simulink model "snap2_f_200msps_64i_4096c"  (R2019a)
settings: Solver=VariableStepDiscrete  StartTime=0.0  StopTime=10.0  RelTol=1e-3
undefined symbols (not defined in the file or in its folder): datetime, posixtime
libraries: xbsIndex_r4 x21354, casper_library_misc x297, casper_library_delays x19, xps_library x14, casper_library_sources x4
(part 5 of 217)

== system snap2_f_200msps_64i_4096c/input ==
  adc : Inport
  noise : Inport  Port=2
  sync : Inport  Port=3
  Constant4 : xbsIndex_r4/Constant  const=0  gui_display_data_type=Fixed-point  arith_type=Unsigned  n_bits=10*64  bin_pt=0  preci_type=Single  exp_width=8  frac_width=24  explicit_period=on  period=1  equ=P=C  opselect=C  inp2=PCIN>>17  opr=+  inp1=P  carry=CIN  dbl_ovrd=off  block_type=constant
  bit_stats : Subsystem
  bus_create2 : Subsystem  AncestorBlock=casper_library_flow_control/bus_create  mask(bus_create){inputNum=4}
      mask prompts: inputNum "Number of inputs:"
      mask init:
      | bus_create_init(gcb,...
      |     'inputNum', inputNum);
  bus_mux : Subsystem  AncestorBlock=casper_library_bus/bus_mux  mask(bus_mux){n_inputs=4, n_bits=10 * ones(64,1), cmplx=off, misc=on, mux_latency=1}
      mask prompts: n_inputs "number of inputs"; n_bits "input bit widths"; cmplx "complex data"; misc "misc support"; mux_latency "mux latency"
      mask help: Mux components of bus
      mask init:
      | bus_mux_init(gcb, ...
      |     'n_inputs', n_inputs, ...
      |     'n_bits', n_bits, ...
      |     'cmplx', cmplx, ...
      |     'misc', misc, ...
      |     'mux_latency', mux_latency);
  counter_test_signal : Subsystem
  rms : Subsystem
  slice3 : xbsIndex_r4/Slice  nbits=2*64  boolean_output=off  mode=Lower Bit Location + Width  bit1=0  base1=MSB of Input  bit0=0  base0=LSB of Input  dbl_ovrd=off  block_type=slice
  source_sel0 : Subsystem  Tag=xps:sw_reg  AncestorBlock=xps_library/Memory/software_register  mask(swreg){io_dir=From Processor, io_delay=0, init_val=0, sample_period=1, names=reg, bitwidths=32, bin_pts=0, arith_types=0, sim_port=on, show_format=off, desc_str=|}
      mask desc_str=|
      | Selector control to determine if signal streams carry
      | ADC samples, digital noise samples, or zeros.
      | Streams ``n=0..15`` is controlled by register
      | bits ``[2n+1:2n]``. Value ``0`` selects noise;
      | ``1`` selects ADC; ``2`` selects zeros.
      mask prompts: io_dir "I/O direction"; io_delay "I/O delay"; init_val "Initial Value"; sample_period "Sample period"; names "Bitfield names [msb...lsb]"; bitwidths "Bitfield widths"; bin_pts "Bitfield binary pts"; arith_types "Bitfield types, ufix=0, fix=1, bool=2"; sim_port "Provide sim input/output?"; show_format "Print format string?"; desc_str "Description"
      mask help: A 32-bit software-accessible register. Can be divided into bitfields of varying widths and types using the fields in the block mask.
      mask init:
      | swreg_init(gcb)
      settings: AttributesFormatString=1input
      mask TypeOptions io_dir: To Processor | From Processor
      mask Callback io_dir:
      | mask_enables = get_param(gcb, 'MaskEnables');
      | mask_names = get_param(gcb, 'MaskNames');
      | if strcmp(get_param(gcb, 'io_dir'), 'To Processor'),
      |     mask_enables{ismember(mask_names, 'sample_period')} = 'off';
      | else
      |     mask_enables{ismember(mask_names, 'sample_period')} = 'on';
      | end
      | set_param(gcb, 'MaskEnables', mask_enables);
      mask DialogControl ParameterTabVar0 Prompt: Setup
  source_sel1 : Subsystem  Tag=xps:sw_reg  AncestorBlock=xps_library/Memory/software_register  mask(swreg){io_dir=From Processor, io_delay=0, init_val=0, sample_period=1, names=reg, bitwidths=32, bin_pts=0, arith_types=0, sim_port=on, show_format=off, desc_str=|}
      mask desc_str=|
      | Selector control to determine if signal streams carry
      | ADC samples, digital noise samples, or zeros.
      | Streams ``n=16..31`` is controlled by register
      | bits ``[2(n-16)+1:2(n-16)]``. Value ``0`` selects noise;
      | ``1`` selects ADC; ``2`` selects zeros.
      mask prompts: io_dir "I/O direction"; io_delay "I/O delay"; init_val "Initial Value"; sample_period "Sample period"; names "Bitfield names [msb...lsb]"; bitwidths "Bitfield widths"; bin_pts "Bitfield binary pts"; arith_types "Bitfield types, ufix=0, fix=1, bool=2"; sim_port "Provide sim input/output?"; show_format "Print format string?"; desc_str "Description"
      mask help: A 32-bit software-accessible register. Can be divided into bitfields of varying widths and types using the fields in the block mask.
      mask init:
      | swreg_init(gcb)
      settings: AttributesFormatString=1input
      mask TypeOptions io_dir: To Processor | From Processor
      mask Callback io_dir:
      | mask_enables = get_param(gcb, 'MaskEnables');
      | mask_names = get_param(gcb, 'MaskNames');
      | if strcmp(get_param(gcb, 'io_dir'), 'To Processor'),
      |     mask_enables{ismember(mask_names, 'sample_period')} = 'off';
      | else
      |     mask_enables{ismember(mask_names, 'sample_period')} = 'on';
      | end
      | set_param(gcb, 'MaskEnables', mask_enables);
      mask DialogControl ParameterTabVar0 Prompt: Setup
  source_sel2 : Subsystem  Tag=xps:sw_reg  AncestorBlock=xps_library/Memory/software_register  mask(swreg){io_dir=From Processor, io_delay=0, init_val=0, sample_period=1, names=reg, bitwidths=32, bin_pts=0, arith_types=0, sim_port=on, show_format=off, desc_str=|}
      mask desc_str=|
      | Selector control to determine if signal streams carry
      | ADC samples, digital noise samples, or zeros.
      | Streams ``n=32..47`` is controlled by register
      | bits ``[2(n-32)+1:2(n-32)]``. Value ``0`` selects noise;
      | ``1`` selects ADC; ``2`` selects zeros.
      mask prompts: io_dir "I/O direction"; io_delay "I/O delay"; init_val "Initial Value"; sample_period "Sample period"; names "Bitfield names [msb...lsb]"; bitwidths "Bitfield widths"; bin_pts "Bitfield binary pts"; arith_types "Bitfield types, ufix=0, fix=1, bool=2"; sim_port "Provide sim input/output?"; show_format "Print format string?"; desc_str "Description"
      mask help: A 32-bit software-accessible register. Can be divided into bitfields of varying widths and types using the fields in the block mask.
      mask init:
      | swreg_init(gcb)
      settings: AttributesFormatString=1input
      mask TypeOptions io_dir: To Processor | From Processor
      mask Callback io_dir:
      | mask_enables = get_param(gcb, 'MaskEnables');
      | mask_names = get_param(gcb, 'MaskNames');
      | if strcmp(get_param(gcb, 'io_dir'), 'To Processor'),
      |     mask_enables{ismember(mask_names, 'sample_period')} = 'off';
      | else
      |     mask_enables{ismember(mask_names, 'sample_period')} = 'on';
      | end
      | set_param(gcb, 'MaskEnables', mask_enables);
      mask DialogControl ParameterTabVar0 Prompt: Setup
  source_sel3 : Subsystem  Tag=xps:sw_reg  AncestorBlock=xps_library/Memory/software_register  mask(swreg){io_dir=From Processor, io_delay=0, init_val=0, sample_period=1, names=reg, bitwidths=32, bin_pts=0, arith_types=0, sim_port=on, show_format=off, desc_str=|}
      mask desc_str=|
      | Selector control to determine if signal streams carry
      | ADC samples, digital noise samples, or zeros.
      | Streams ``n=48..63`` is controlled by register
      | bits ``[2(n-48)+1:2(n-48)]``. Value ``0`` selects noise;
      | ``1`` selects ADC; ``2`` selects zeros.
      mask prompts: io_dir "I/O direction"; io_delay "I/O delay"; init_val "Initial Value"; sample_period "Sample period"; names "Bitfield names [msb...lsb]"; bitwidths "Bitfield widths"; bin_pts "Bitfield binary pts"; arith_types "Bitfield types, ufix=0, fix=1, bool=2"; sim_port "Provide sim input/output?"; show_format "Print format string?"; desc_str "Description"
      mask help: A 32-bit software-accessible register. Can be divided into bitfields of varying widths and types using the fields in the block mask.
      mask init:
      | swreg_init(gcb)
      settings: AttributesFormatString=1input
      mask TypeOptions io_dir: To Processor | From Processor
      mask Callback io_dir:
      | mask_enables = get_param(gcb, 'MaskEnables');
      | mask_names = get_param(gcb, 'MaskNames');
      | if strcmp(get_param(gcb, 'io_dir'), 'To Processor'),
      |     mask_enables{ismember(mask_names, 'sample_period')} = 'off';
      | else
      |     mask_enables{ismember(mask_names, 'sample_period')} = 'on';
      | end
      | set_param(gcb, 'MaskEnables', mask_enables);
      mask DialogControl ParameterTabVar0 Prompt: Setup
  sync_out : Outport
  dout : Outport  Port=2
  wires:
  Constant4/1 -> bus_mux/4(d2)
  sync/1 -> bus_mux/6(misci)
  bus_mux/1(out) -> dout/1, bit_stats/1(din), rms/1(in)
  slice3/1 -> bus_mux/1(sel)
  adc/1 -> bus_mux/3(d1)
  noise/1 -> bus_mux/2(d0)
  bus_mux/2(misco) -> sync_out/1
  source_sel1/1(in_reg) -> bus_create2/2(in2)
  source_sel0/1(in_reg) -> bus_create2/1(in1)
  source_sel2/1(in_reg) -> bus_create2/3(in3)
  bus_create2/1(bus_out) -> slice3/1
  source_sel3/1(in_reg) -> bus_create2/4(in4)
  counter_test_signal/1(Out1) -> bus_mux/5(d3)

== system snap2_f_200msps_64i_4096c/mask ==
  note: accumulation length in spectra
  note: delay by 2 so new_acc precedes
      | first spectra of a new accumulation.
      | 1 cycle for tt_counter load.
      | 1 cycle for target_tt compare
  note: starts on 1
  sync : Inport
  din : Inport  Port=2
  tt : Inport  Port=3
  Concat : xbsIndex_r4/Concat  num_inputs=2  dbl_ovrd=off  block_type=concat
  Constant : Constant  Value=8192*2
  Constant1 : Constant  Value=0
  Constant2 : Constant  Value=3
  Constant3 : Constant  Value=10
  Counter : xbsIndex_r4/Counter  cnt_type=Free Running  cnt_to=Inf  operation=Up  start_count=1  cnt_by_val=1  arith_type=Unsigned  n_bits=32  bin_pt=0  load_pin=off  rst=on  en=off  explicit_period=on  period=1  use_behavioral_HDL=off  implementation=Fabric  dbl_ovrd=off  block_type=counter
  Counter1 : xbsIndex_r4/Counter  cnt_type=Free Running  cnt_to=Inf  operation=Up  start_count=0  cnt_by_val=1  arith_type=Unsigned  n_bits=32  bin_pt=0  load_pin=off  rst=off  en=on  explicit_period=on  period=1  use_behavioral_HDL=off  implementation=Fabric  dbl_ovrd=off  block_type=counter
  Delay{,1..7} (8 alike) : xbsIndex_r4/Delay  rst=off  infoeditControl=Selection of Reset will increase slice count due to use of real FFs and instead of SRLs  en=off  latency=2  reg_retiming=on  dbl_ovrd=off  block_type=delay
  Delay8 : xbsIndex_r4/Delay  rst=off  infoeditControl=Selection of Reset will increase slice count due to use of real FFs and instead of SRLs  en=off  latency=1  reg_retiming=on  dbl_ovrd=off  block_type=delay
  Logical : xbsIndex_r4/Logical  logical_function=OR  inputs=2  en=off  latency=0  precision=Full  arith_type=Unsigned  n_bits=16  bin_pt=0  align_bp=on  dbl_ovrd=off  block_type=logical
  Register : xbsIndex_r4/Register  init=0  rst=off  en=on  dbl_ovrd=off  block_type=register
  Reinterpret : xbsIndex_r4/Reinterpret  force_arith_type=off  arith_type=Unsigned  force_bin_pt=on  bin_pt=18  block_type=reinterpret
  Relational : xbsIndex_r4/Relational  mode=a=b  op_type=Bool  en=off  latency=1  dbl_ovrd=off  block_type=relational
  Relational1 : xbsIndex_r4/Relational  mode=a=b  op_type=Bool  en=off  latency=0  dbl_ovrd=off  block_type=relational
  Slice : xbsIndex_r4/Slice  nbits=32-(nfft_bits - 3 + ninput_bits - 2)  boolean_output=off  mode=Lower Bit Location + Width  bit1=0  base1=MSB of Input  bit0=nfft_bits - 3 + ninput_bits - 2  base0=LSB of Input  dbl_ovrd=off  block_type=slice
  acc_cnt : Subsystem  Tag=xps:sw_reg  AncestorBlock=xps_library/Memory/software_register  mask(swreg){io_dir=To Processor, io_delay=0, init_val=0, sample_period=1, names=reg, bitwidths=32, bin_pts=0, arith_types=0, sim_port=on, show_format=on, desc_str=""}
      mask prompts: io_dir "I/O direction"; io_delay "I/O delay"; init_val "Initial Value"; sample_period "Sample period"; names "Bitfield names [msb...lsb]"; bitwidths "Bitfield widths"; bin_pts "Bitfield binary pts"; arith_types "Bitfield types, ufix=0, fix=1, bool=2"; sim_port "Provide sim input/output?"; show_format "Print format string?"; desc_str "Description"
      mask help: A 32-bit software-accessible register. Can be divided into bitfields of varying widths and types using the fields in the block mask.
      mask init:
      | swreg_init(gcb)
      settings: AttributesFormatString=1output:uf32.0 = 32 bits
      mask TypeOptions io_dir: To Processor | From Processor
      mask Callback io_dir:
      | mask_enables = get_param(gcb, 'MaskEnables');
      | mask_names = get_param(gcb, 'MaskNames');
      | if strcmp(get_param(gcb, 'io_dir'), 'To Processor'),
      |     mask_enables{ismember(mask_names, 'sample_period')} = 'off';
      | else
      |     mask_enables{ismember(mask_names, 'sample_period')} = 'on';
      | end
      | set_param(gcb, 'MaskEnables', mask_enables);
      mask DialogControl ParameterTabVar0 Prompt: Setup
  acc_len : Subsystem  Tag=xps:sw_reg  AncestorBlock=xps_library/Memory/software_register  mask(swreg){io_dir=From Processor, io_delay=0, init_val=0, sample_period=1, names=reg, bitwidths=32, bin_pts=0, arith_types=0, sim_port=on, show_format=on, desc_str=""}
      mask prompts: io_dir "I/O direction"; io_delay "I/O delay"; init_val "Initial Value"; sample_period "Sample period"; names "Bitfield names [msb...lsb]"; bitwidths "Bitfield widths"; bin_pts "Bitfield binary pts"; arith_types "Bitfield types, ufix=0, fix=1, bool=2"; sim_port "Provide sim input/output?"; show_format "Print format string?"; desc_str "Description"
      mask help: A 32-bit software-accessible register. Can be divided into bitfields of varying widths and types using the fields in the block mask.
      mask init:
      | swreg_init(gcb)
      settings: AttributesFormatString=1input:uf32.0 = 32 bits
      mask TypeOptions io_dir: To Processor | From Processor
      mask Callback io_dir:
      | mask_enables = get_param(gcb, 'MaskEnables');
      | mask_names = get_param(gcb, 'MaskNames');
      | if strcmp(get_param(gcb, 'io_dir'), 'To Processor'),
      |     mask_enables{ismember(mask_names, 'sample_period')} = 'off';
      | else
      |     mask_enables{ismember(mask_names, 'sample_period')} = 'on';
      | end
      | set_param(gcb, 'MaskEnables', mask_enables);
      mask DialogControl ParameterTabVar0 Prompt: Setup
  acc_time_lsb : Subsystem  Tag=xps:sw_reg  AncestorBlock=xps_library/Memory/software_register  mask(swreg){io_dir=To Processor, io_delay=0, init_val=0, sample_period=1, names=reg, bitwidths=32, bin_pts=0, arith_types=0, sim_port=on, show_format=on, desc_str=""}
      mask prompts: io_dir "I/O direction"; io_delay "I/O delay"; init_val "Initial Value"; sample_period "Sample period"; names "Bitfield names [msb...lsb]"; bitwidths "Bitfield widths"; bin_pts "Bitfield binary pts"; arith_types "Bitfield types, ufix=0, fix=1, bool=2"; sim_port "Provide sim input/output?"; show_format "Print format string?"; desc_str "Description"
      mask help: A 32-bit software-accessible register. Can be divided into bitfields of varying widths and types using the fields in the block mask.
      mask init:
      | swreg_init(gcb)
      settings: AttributesFormatString=1output:uf32.0 = 32 bits
      mask TypeOptions io_dir: To Processor | From Processor
      mask Callback io_dir:
      | mask_enables = get_param(gcb, 'MaskEnables');
      | mask_names = get_param(gcb, 'MaskNames');
      | if strcmp(get_param(gcb, 'io_dir'), 'To Processor'),
      |     mask_enables{ismember(mask_names, 'sample_period')} = 'off';
      | else
      |     mask_enables{ismember(mask_names, 'sample_period')} = 'on';
      | end
      | set_param(gcb, 'MaskEnables', mask_enables);
      mask DialogControl ParameterTabVar0 Prompt: Setup
  acc_time_msb : Subsystem  Tag=xps:sw_reg  AncestorBlock=xps_library/Memory/software_register  mask(swreg){io_dir=To Processor, io_delay=0, init_val=0, sample_period=1, names=reg, bitwidths=32, bin_pts=0, arith_types=0, sim_port=on, show_format=on, desc_str=""}
      mask prompts: io_dir "I/O direction"; io_delay "I/O delay"; init_val "Initial Value"; sample_period "Sample period"; names "Bitfield names [msb...lsb]"; bitwidths "Bitfield widths"; bin_pts "Bitfield binary pts"; arith_types "Bitfield types, ufix=0, fix=1, bool=2"; sim_port "Provide sim input/output?"; show_format "Print format string?"; desc_str "Description"
      mask help: A 32-bit software-accessible register. Can be divided into bitfields of varying widths and types using the fields in the block mask.
      mask init:
      | swreg_init(gcb)
      settings: AttributesFormatString=1output:uf32.0 = 32 bits
      mask TypeOptions io_dir: To Processor | From Processor
      mask Callback io_dir:
      | mask_enables = get_param(gcb, 'MaskEnables');
      | mask_names = get_param(gcb, 'MaskNames');
      | if strcmp(get_param(gcb, 'io_dir'), 'To Processor'),
      |     mask_enables{ismember(mask_names, 'sample_period')} = 'off';
      | else
      |     mask_enables{ismember(mask_names, 'sample_period')} = 'on';
      | end
      | set_param(gcb, 'MaskEnables', mask_enables);
      mask DialogControl ParameterTabVar0 Prompt: Setup
  bus_create2 : Subsystem  AncestorBlock=casper_library_flow_control/bus_create  mask(bus_create){inputNum=4}
      mask prompts: inputNum "Number of inputs:"
      mask init:
      | bus_create_init(gcb,...
      |     'inputNum', inputNum);
  bus_expand : Subsystem  AncestorBlock=casper_library_flow_control/bus_expand  mask(bus_expand){mode=divisions of equal size, outputNum=2, outputWidth=32, outputBinaryPt=0, outputArithmeticType=0, show_format=off, outputToWorkspace=off, variablePrefix=out, outputToModelAsWell=on}
      mask prompts: outputNum "Number of outputs:"; outputWidth "Output width:"; outputBinaryPt "Output binary point position:"; outputArithmeticType "Output arithmetic type (ufix=0, fix=1, bool=2):"; show_format "Print format string?"; outputToWorkspace "Output to workspace?"; variablePrefix "Variable name prefix:"; outputToModelAsWell "Output to model as well?"
      mask help:
      | Expands a 'bus' made using a bus_create or Xilinx
      | concat block.
      | The input will be divided into the specified number
      | of outputs with the specified arithmetic types.
      | Divisions are made from most significant bit.
      mask init: same as snap2_f_200msps_64i_4096c/autocorr/bus_expand
      settings: AttributesFormatString=2 outputs
      mask TypeOptions mode: divisions of equal size | divisions of arbitrary size
      mask Callback mode: bus_expand_callback();
      mask Callback outputWidth: bus_expand_callback();
      mask Callback outputToWorkspace: bus_expand_callback();
  bus_expand4 : Subsystem  AncestorBlock=casper_library_flow_control/bus_expand  mask(bus_expand){mode=divisions of equal size, outputNum=4, outputWidth=36*8, outputBinaryPt=0, outputArithmeticType=0, show_format=off, outputToWorkspace=off, variablePrefix=out, outputToModelAsWell=on}
      mask prompts: outputNum "Number of outputs:"; outputWidth "Output width:"; outputBinaryPt "Output binary point position:"; outputArithmeticType "Output arithmetic type (ufix=0, fix=1, bool=2):"; show_format "Print format string?"; outputToWorkspace "Output to workspace?"; variablePrefix "Variable name prefix:"; outputToModelAsWell "Output to model as well?"
      mask help:
      | Expands a 'bus' made using a bus_create or Xilinx
      | concat block.
      | The input will be divided into the specified number
      | of outputs with the specified arithmetic types.
      | Divisions are made from most significant bit.
      mask init: same as snap2_f_200msps_64i_4096c/autocorr/bus_expand
      settings: AttributesFormatString=4 outputs
      mask TypeOptions mode: divisions of equal size | divisions of arbitrary size
      mask Callback mode: bus_expand_callback();
      mask Callback outputWidth: bus_expand_callback();
      mask Callback outputToWorkspace: bus_expand_callback();
  core0 : Subsystem  mask{nchan_bits=nfft_bits - 3, ninput_bits=ninput_bits - 2, ram_latency=2}
      mask prompts: nchan_bits "Number of fft channels (2^?)"; ninput_bits "Number of Input signals (2^?)"; ram_latency "RAM latency"
  core1 : Subsystem  mask{nchan_bits=nfft_bits - 3, ninput_bits=ninput_bits - 2, ram_latency=2}
      mask prompts: nchan_bits "Number of fft channels (2^?)"; ninput_bits "Number of Input signals (2^?)"; ram_latency "RAM latency"
  core2 : Subsystem  mask{nchan_bits=nfft_bits - 3, ninput_bits=ninput_bits - 2, ram_latency=2}
      mask prompts: nchan_bits "Number of fft channels (2^?)"; ninput_bits "Number of Input signals (2^?)"; ram_latency "RAM latency"
  core3 : Subsystem  mask{nchan_bits=nfft_bits - 3, ninput_bits=ninput_bits - 2, ram_latency=2}
      mask prompts: nchan_bits "Number of fft channels (2^?)"; ninput_bits "Number of Input signals (2^?)"; ram_latency "RAM latency"
  target_tt_lsb : Subsystem  Tag=xps:sw_reg  AncestorBlock=xps_library/Memory/software_register  mask(swreg){io_dir=From Processor, io_delay=0, init_val=0, sample_period=1, names=reg, bitwidths=32, bin_pts=0, arith_types=0, sim_port=on, show_format=on, desc_str=""}
      mask prompts: io_dir "I/O direction"; io_delay "I/O delay"; init_val "Initial Value"; sample_period "Sample period"; names "Bitfield names [msb...lsb]"; bitwidths "Bitfield widths"; bin_pts "Bitfield binary pts"; arith_types "Bitfield types, ufix=0, fix=1, bool=2"; sim_port "Provide sim input/output?"; show_format "Print format string?"; desc_str "Description"
      mask help: A 32-bit software-accessible register. Can be divided into bitfields of varying widths and types using the fields in the block mask.
      mask init:
      | swreg_init(gcb)
      settings: AttributesFormatString=1input:uf32.0 = 32 bits
      mask TypeOptions io_dir: To Processor | From Processor
      mask Callback io_dir:
      | mask_enables = get_param(gcb, 'MaskEnables');
      | mask_names = get_param(gcb, 'MaskNames');
      | if strcmp(get_param(gcb, 'io_dir'), 'To Processor'),
      |     mask_enables{ismember(mask_names, 'sample_period')} = 'off';
      | else
      |     mask_enables{ismember(mask_names, 'sample_period')} = 'on';
      | end
      | set_param(gcb, 'MaskEnables', mask_enables);
      mask DialogControl ParameterTabVar0 Prompt: Setup
  target_tt_msb : Subsystem  Tag=xps:sw_reg  AncestorBlock=xps_library/Memory/software_register  mask(swreg){io_dir=From Processor, io_delay=0, init_val=0, sample_period=1, names=reg, bitwidths=32, bin_pts=0, arith_types=0, sim_port=on, show_format=on, desc_str=""}
      mask prompts: io_dir "I/O direction"; io_delay "I/O delay"; init_val "Initial Value"; sample_period "Sample period"; names "Bitfield names [msb...lsb]"; bitwidths "Bitfield widths"; bin_pts "Bitfield binary pts"; arith_types "Bitfield types, ufix=0, fix=1, bool=2"; sim_port "Provide sim input/output?"; show_format "Print format string?"; desc_str "Description"
      mask help: A 32-bit software-accessible register. Can be divided into bitfields of varying widths and types using the fields in the block mask.
      mask init:
      | swreg_init(gcb)
      settings: AttributesFormatString=1input:uf32.0 = 32 bits
      mask TypeOptions io_dir: To Processor | From Processor
      mask Callback io_dir:
      | mask_enables = get_param(gcb, 'MaskEnables');
      | mask_names = get_param(gcb, 'MaskNames');
      | if strcmp(get_param(gcb, 'io_dir'), 'To Processor'),
      |     mask_enables{ismember(mask_names, 'sample_period')} = 'off';
      | else
      |     mask_enables{ismember(mask_names, 'sample_period')} = 'on';
      | end
      | set_param(gcb, 'MaskEnables', mask_enables);
      mask DialogControl ParameterTabVar0 Prompt: Setup
  threshold : Subsystem  Tag=xps:sw_reg  AncestorBlock=xps_library/Memory/software_register  mask(swreg){io_dir=From Processor, io_delay=0, init_val=2^32 - 1, sample_period=1, names=reg, bitwidths=32, bin_pts=0, arith_types=0, sim_port=on, show_format=on, desc_str=""}
      mask prompts: io_dir "I/O direction"; io_delay "I/O delay"; init_val "Initial Value"; sample_period "Sample period"; names "Bitfield names [msb...lsb]"; bitwidths "Bitfield widths"; bin_pts "Bitfield binary pts"; arith_types "Bitfield types, ufix=0, fix=1, bool=2"; sim_port "Provide sim input/output?"; show_format "Print format string?"; desc_str "Description"
      mask help: A 32-bit software-accessible register. Can be divided into bitfields of varying widths and types using the fields in the block mask.
      mask init:
      | swreg_init(gcb)
      settings: AttributesFormatString=1input:uf32.0 = 32 bits
      mask TypeOptions io_dir: To Processor | From Processor
      mask Callback io_dir:
      | mask_enables = get_param(gcb, 'MaskEnables');
      | mask_names = get_param(gcb, 'MaskNames');
      | if strcmp(get_param(gcb, 'io_dir'), 'To Processor'),
      |     mask_enables{ismember(mask_names, 'sample_period')} = 'off';
      | else
      |     mask_enables{ismember(mask_names, 'sample_period')} = 'on';
      | end
      | set_param(gcb, 'MaskEnables', mask_enables);
      mask DialogControl ParameterTabVar0 Prompt: Setup
  tt_counter : xbsIndex_r4/Counter  cnt_type=Free Running  cnt_to=1  operation=Up  start_count=0  cnt_by_val=1  arith_type=Unsigned  n_bits=64  bin_pt=0  load_pin=on  rst=off  en=off  explicit_period=on  period=1  use_behavioral_HDL=off  implementation=Fabric  use_rpm=on  dbl_ovrd=off  block_type=counter
      settings: xl_area=[0, 0, 0, 0, 0, 0, 0]
  sync_out : Outport
  dout : Outport  Port=2
  wires:
  bus_create2/1(bus_out) -> dout/1
  core0/2(dout) -> bus_create2/1(in1)
  bus_expand4/1(msb_out4) -> Delay1/1
  [sync_in] -> Delay/1
  sync/1 -> tt_counter/1, [sync_in]
  din/1 -> bus_expand4/1(bus_in)
  core0/1(sync_out) -> sync_out/1
  tt/1 -> tt_counter/2
  tt_counter/1 -> Relational/2, Delay8/1
  target_tt_lsb/1(in_reg) -> Concat/2
  target_tt_msb/1(in_reg) -> Concat/1
  Concat/1 -> Relational/1
  Counter/1 -> Slice/1
  Slice/1 -> Relational1/1
  acc_len/1(in_reg) -> Relational1/2
  Logical/1 -> [new_acc], Counter/1
  Relational/1 -> Logical/2
  Relational1/1 -> Logical/1, Register/2, Counter1/1
  Counter1/1 -> acc_cnt/1(out_reg)
  Constant/1 -> target_tt_lsb/1(sim_1)
  Constant1/1 -> target_tt_msb/1(sim_1)
  Constant2/1 -> acc_len/1(sim_1)
  Constant3/1 -> threshold/1(sim_1)
  threshold/1(in_reg) -> Reinterpret/1
  Reinterpret/1 -> [threshold]
  [sync_in] -> Delay2/1
  bus_expand4/2(out3) -> Delay3/1
  bus_expand4/3(out2) -> Delay5/1
  [sync_in] -> Delay4/1
  [sync_in] -> Delay6/1
  bus_expand4/4(lsb_out1) -> Delay7/1
  core1/2(dout) -> bus_create2/2(in2)
  core2/2(dout) -> bus_create2/3(in3)
  core3/2(dout) -> bus_create2/4(in4)
  Delay8/1 -> Register/1
  Register/1 -> bus_expand/1(bus_in)
  bus_expand/1(msb_out2) -> acc_time_msb/1(out_reg)
  bus_expand/2(lsb_out1) -> acc_time_lsb/1(out_reg)
  Delay/1 -> core0/1(sync)
  [new_acc] -> core0/3(new_acc)
  [new_acc] -> core1/3(new_acc)
  Delay2/1 -> core1/1(sync)
  [new_acc] -> core2/3(new_acc)
  [new_acc] -> core3/3(new_acc)
  Delay3/1 -> core1/2(in)
  Delay4/1 -> core2/1(sync)
  Delay5/1 -> core2/2(in)
  Delay6/1 -> core3/1(sync)
  Delay7/1 -> core3/2(in)
  Delay1/1 -> core0/2(in)

== system snap2_f_200msps_64i_4096c/noise ==
  sync_in : Inport
  arm_noise : Inport  Port=2
  BitBasher : xbsIndex_r4/BitBasher  bitexpr=|  display_expr=off  sr_1=1  arith_type1=Unsigned  bin_pt1=0  sr_2=2  arith_type2=Unsigned  bin_pt2=0  sr_3=3  arith_type3=Unsigned  bin_pt3=0  sr_4=4  arith_type4=Unsigned  bin_pt4=0  dbl_ovrd=off  block_type=bitbasher
      | <!DOCTYPE HTML PUBLIC "-//W3C//DTD HTML 4.0//EN" "http://www.w3.org/TR/REC-html40/strict.dtd">
      | <html><head><meta name="qrichtext" content="1" /><style type="text/css">
      | p, li { white-space: pre-wrap; }
      | </style></head><body style=" font-family:'Sans'; font-size:10pt; font-weight:400; font-style:normal;">
      | <p style=" margin-top:12px; margin-bottom:12px; margin-left:0px; margin-right:0px; -qt-block-indent:0; text-indent:0px;"><span style=" font-family:'MS Shell Dlg'; font-size:8pt;">s0={8'h5c, s32[7:0], s32[0:7], 8'ha3}<br />s1={8'h5c, s32[15:8], s32[8:15], 8'ha3}<br />s2={8'h5c, s32[23:16], s32[16:23], 8'ha3}<br />s3={8'h5c, s32[31:24], s32[24:31], 8'ha3}</span></p></body></html>
  Constant : Constant  Value=0
  Delay{,1..7} (8 alike) : xbsIndex_r4/Delay  rst=off  infoeditControl=Selection of Reset will increase slice count due to use of real FFs and instead of SRLs  en=off  latency=1  reg_retiming=off  dbl_ovrd=off  block_type=delay
  From2 : From  Commented=on  GotoTag=seed2
      settings: CloseFcn=tagdialog Close
  From3 : From  Commented=on  GotoTag=seed3
      settings: CloseFcn=tagdialog Close
  From6 : From  Commented=on  GotoTag=seed_ld
      settings: CloseFcn=tagdialog Close
  From7 : From  Commented=on  GotoTag=seed_ld
      settings: CloseFcn=tagdialog Close
  From71 : From  Commented=on  GotoTag=noise0
  From72 : From  Commented=on  GotoTag=noise4
  From73 : From  Commented=on  GotoTag=noise5
  From74 : From  Commented=on  GotoTag=noise6
  From75 : From  Commented=on  GotoTag=noise7
  From76 : From  Commented=on  GotoTag=noise3
  From77 : From  Commented=on  GotoTag=noise1
  From78 : From  Commented=on  GotoTag=noise2
  Goto_noise4 : Goto  Commented=on  GotoTag=noise4
  Goto_noise5 : Goto  Commented=on  GotoTag=noise5
  Goto_noise6 : Goto  Commented=on  GotoTag=noise6
  Goto_noise7 : Goto  Commented=on  GotoTag=noise7
  armed_trigger : casper_library_misc/armed_trigger
      settings: SourceProductName=CASPER DSP Blockset
  bus_create1 : Subsystem  AncestorBlock=casper_library_flow_control/bus_create  mask(bus_create){inputNum=8}
      mask prompts: inputNum "Number of inputs:"
      mask init:
      | bus_create_init(gcb,...
      |     'inputNum', inputNum);
  bus_create10 : Subsystem  Commented=on  AncestorBlock=casper_library_flow_control/bus_create  mask(bus_create){inputNum=8}
      mask prompts: inputNum "Number of inputs:"
      mask init:
      | bus_create_init(gcb,...
      |     'inputNum', inputNum);
  bus_create2 : Subsystem  AncestorBlock=casper_library_flow_control/bus_create  mask(bus_create){inputNum=8}
      mask prompts: inputNum "Number of inputs:"
      mask init:
      | bus_create_init(gcb,...
      |     'inputNum', inputNum);
  bus_create3 : Subsystem  AncestorBlock=casper_library_flow_control/bus_create  mask(bus_create){inputNum=8}
      mask prompts: inputNum "Number of inputs:"
      mask init:
      | bus_create_init(gcb,...
      |     'inputNum', inputNum);
  bus_create4 : Subsystem  AncestorBlock=casper_library_flow_control/bus_create  mask(bus_create){inputNum=8}
      mask prompts: inputNum "Number of inputs:"
      mask init:
      | bus_create_init(gcb,...
      |     'inputNum', inputNum);
  bus_create5 : Subsystem  AncestorBlock=casper_library_flow_control/bus_create  mask(bus_create){inputNum=8}
      mask prompts: inputNum "Number of inputs:"
      mask init:
      | bus_create_init(gcb,...
      |     'inputNum', inputNum);
  bus_create6 : Subsystem  AncestorBlock=casper_library_flow_control/bus_create  mask(bus_create){inputNum=8}
      mask prompts: inputNum "Number of inputs:"
      mask init:
      | bus_create_init(gcb,...
      |     'inputNum', inputNum);
  bus_create7 : Subsystem  AncestorBlock=casper_library_flow_control/bus_create  mask(bus_create){inputNum=8}
      mask prompts: inputNum "Number of inputs:"
      mask init:
      | bus_create_init(gcb,...
      |     'inputNum', inputNum);
  bus_create8 : Subsystem  AncestorBlock=casper_library_flow_control/bus_create  mask(bus_create){inputNum=8}
      mask prompts: inputNum "Number of inputs:"
      mask init:
      | bus_create_init(gcb,...
      |     'inputNum', inputNum);
  bus_create9 : Subsystem  AncestorBlock=casper_library_flow_control/bus_create  mask(bus_create){inputNum=8}
      mask prompts: inputNum "Number of inputs:"
      mask init:
      | bus_create_init(gcb,...
      |     'inputNum', inputNum);
  noise0 : Subsystem
  noise1 : Subsystem
  noise2 : Subsystem  Commented=on
  noise3 : Subsystem  Commented=on
  octal_mux0 : Subsystem
  octal_mux1 : Subsystem
  octal_mux2 : Subsystem
  octal_mux3 : Subsystem
  octal_mux4 : Subsystem
  octal_mux5 : Subsystem
  octal_mux6 : Subsystem
  octal_mux7 : Subsystem
  octal_mux8 : Subsystem  Commented=on
  seeds0 : Subsystem  Tag=xps:sw_reg  AncestorBlock=xps_library/Memory/software_register  mask(swreg){io_dir=From Processor, io_delay=0, init_val=0, sample_period=1, names=reg, bitwidths=32, bin_pts=0, arith_types=0, sim_port=on, show_format=off, desc_str=|}
      mask desc_str=|
      | Noise generator seed values. If the 32-bit value in this
      | register is ``v``, the seed for the first
      | noise generator is (using Verilog syntax)
      | ``{8'h5c, v[7:0], v[0:7], 8'ha3}``.
      | The seed for the second noise generator is
      | ``{8'h5c, v[15:8], v[8:15], 8'ha3}``.
      | The seed for the third noise generator is
      | ``{8'h5c, v[23:16], v[16:23], 8'ha3}``.
      | The seed for the fourth noise generator is
      | ``{8'h5c, v[31:24], v[24:31], 8'ha3}``
      mask prompts: io_dir "I/O direction"; io_delay "I/O delay"; init_val "Initial Value"; sample_period "Sample period"; names "Bitfield names [msb...lsb]"; bitwidths "Bitfield widths"; bin_pts "Bitfield binary pts"; arith_types "Bitfield types, ufix=0, fix=1, bool=2"; sim_port "Provide sim input/output?"; show_format "Print format string?"; desc_str "Description"
      mask help: A 32-bit software-accessible register. Can be divided into bitfields of varying widths and types using the fields in the block mask.
      mask init:
      | swreg_init(gcb)
      settings: AttributesFormatString=1input
      mask TypeOptions io_dir: To Processor | From Processor
      mask Callback io_dir:
      | mask_enables = get_param(gcb, 'MaskEnables');
      | mask_names = get_param(gcb, 'MaskNames');
      | if strcmp(get_param(gcb, 'io_dir'), 'To Processor'),
      |     mask_enables{ismember(mask_names, 'sample_period')} = 'off';
      | else
      |     mask_enables{ismember(mask_names, 'sample_period')} = 'on';
      | end
      | set_param(gcb, 'MaskEnables', mask_enables);
      mask DialogControl ParameterTabVar0 Prompt: Setup
  noise : Outport
  seed_ld : Outport  Port=2
  wires:
  [seed0] -> noise0/1(seed)
  From3/1 -> noise3/1(seed)
  From2/1 -> noise2/1(seed)
  [seed1] -> noise1/1(seed)
  From7/1 -> noise3/2(ld)
  From6/1 -> noise2/2(ld)
  [seed_ld] -> noise1/2(ld)
  [seed_ld] -> noise0/2(ld)
  bus_create5/1(bus_out) -> noise/1
  noise0/1(n1) -> [noise0]  "n0"
  noise1/2(n2) -> [noise3]  "n1"
  BitBasher/2 -> [seed1]
  seeds0/1(in_reg) -> BitBasher/1
  BitBasher/3 -> [seed2]
  Constant/1 -> seeds0/1(sim_1)
  BitBasher/1 -> [seed0]
  BitBasher/4 -> [seed3]
  sync_in/1 -> armed_trigger/2
  armed_trigger/1 -> [seed_ld], seed_ld/1
  arm_noise/1 -> armed_trigger/1
  noise0/2(n2) -> [noise1]  "n1"
  noise1/1(n1) -> [noise2]  "n0"
  noise2/1(n1) -> Goto_noise4/1  "n0"
  noise2/2(n2) -> Goto_noise5/1  "n1"
  noise3/1(n1) -> Goto_noise6/1  "n0"
  noise3/2(n2) -> Goto_noise7/1  "n1"
  [noise0] -> octal_mux0/1(n0)
  [noise1] -> octal_mux0/2(n1)
  [noise2] -> octal_mux0/3(n2)
  [noise3] -> octal_mux0/4(n3)
  octal_mux0/1(out0) -> bus_create1/1(in1)
  octal_mux0/2(out1) -> bus_create1/2(in2)
  octal_mux0/3(out2) -> bus_create1/3(in3)
  octal_mux0/4(out3) -> bus_create1/4(in4)
  octal_mux0/5(out4) -> bus_create1/5(in5)
  octal_mux0/6(out5) -> bus_create1/6(in6)
  octal_mux0/7(out6) -> bus_create1/7(in7)
  octal_mux0/8(out7) -> bus_create1/8(in8)
  Delay/1 -> bus_create5/1(in1)
  Delay1/1 -> bus_create5/2(in2)
  Delay2/1 -> bus_create5/3(in3)
  Delay3/1 -> bus_create5/4(in4)
  Delay4/1 -> bus_create5/5(in5)
  Delay5/1 -> bus_create5/6(in6)
  Delay6/1 -> bus_create5/7(in7)
  Delay7/1 -> bus_create5/8(in8)
  bus_create1/1(bus_out) -> Delay/1
  bus_create2/1(bus_out) -> Delay1/1
  bus_create3/1(bus_out) -> Delay2/1
  bus_create4/1(bus_out) -> Delay3/1
  bus_create6/1(bus_out) -> Delay4/1
  bus_create7/1(bus_out) -> Delay5/1
  bus_create8/1(bus_out) -> Delay6/1
  bus_create9/1(bus_out) -> Delay7/1
  octal_mux8/8(out7) -> bus_create10/8(in8)
  octal_mux8/7(out6) -> bus_create10/7(in7)
  octal_mux8/6(out5) -> bus_create10/6(in6)
  octal_mux8/5(out4) -> bus_create10/5(in5)
  octal_mux8/4(out3) -> bus_create10/4(in4)
  octal_mux8/3(out2) -> bus_create10/3(in3)
  octal_mux8/2(out1) -> bus_create10/2(in2)
  octal_mux8/1(out0) -> bus_create10/1(in1)
  From75/1 -> octal_mux8/8(n7)
  From74/1 -> octal_mux8/7(n6)
  From73/1 -> octal_mux8/6(n5)
  From72/1 -> octal_mux8/5(n4)
  From76/1 -> octal_mux8/4(n3)
  From78/1 -> octal_mux8/3(n2)
  From77/1 -> octal_mux8/2(n1)
  From71/1 -> octal_mux8/1(n0)
  octal_mux1/8(out7) -> bus_create2/8(in8)
  octal_mux1/7(out6) -> bus_create2/7(in7)
  octal_mux1/6(out5) -> bus_create2/6(in6)
  octal_mux1/5(out4) -> bus_create2/5(in5)
  octal_mux1/4(out3) -> bus_create2/4(in4)
  octal_mux1/3(out2) -> bus_create2/3(in3)
  octal_mux1/2(out1) -> bus_create2/2(in2)
  octal_mux1/1(out0) -> bus_create2/1(in1)
  [noise3] -> octal_mux1/4(n3)
  [noise2] -> octal_mux1/3(n2)
  [noise1] -> octal_mux1/2(n1)
  [noise0] -> octal_mux1/1(n0)
  [noise0] -> octal_mux2/1(n0)
  [noise1] -> octal_mux2/2(n1)
  [noise2] -> octal_mux2/3(n2)
  [noise3] -> octal_mux2/4(n3)
  octal_mux2/1(out0) -> bus_create3/1(in1)
  octal_mux2/2(out1) -> bus_create3/2(in2)
  octal_mux2/3(out2) -> bus_create3/3(in3)
  octal_mux2/4(out3) -> bus_create3/4(in4)
  octal_mux2/5(out4) -> bus_create3/5(in5)
  octal_mux2/6(out5) -> bus_create3/6(in6)
  octal_mux2/7(out6) -> bus_create3/7(in7)
  octal_mux2/8(out7) -> bus_create3/8(in8)
  octal_mux3/8(out7) -> bus_create4/8(in8)
  octal_mux3/7(out6) -> bus_create4/7(in7)
  octal_mux3/6(out5) -> bus_create4/6(in6)
  octal_mux3/5(out4) -> bus_create4/5(in5)
  octal_mux3/4(out3) -> bus_create4/4(in4)
  octal_mux3/3(out2) -> bus_create4/3(in3)
  octal_mux3/2(out1) -> bus_create4/2(in2)
  octal_mux3/1(out0) -> bus_create4/1(in1)
  [noise3] -> octal_mux3/4(n3)
  [noise2] -> octal_mux3/3(n2)
  [noise1] -> octal_mux3/2(n1)
  [noise0] -> octal_mux3/1(n0)
  [noise0] -> octal_mux4/1(n0)
  [noise1] -> octal_mux4/2(n1)
  [noise2] -> octal_mux4/3(n2)
  [noise3] -> octal_mux4/4(n3)
  octal_mux4/1(out0) -> bus_create6/1(in1)
  octal_mux4/2(out1) -> bus_create6/2(in2)
  octal_mux4/3(out2) -> bus_create6/3(in3)
  octal_mux4/4(out3) -> bus_create6/4(in4)
  octal_mux4/5(out4) -> bus_create6/5(in5)
  octal_mux4/6(out5) -> bus_create6/6(in6)
  octal_mux4/7(out6) -> bus_create6/7(in7)
  octal_mux4/8(out7) -> bus_create6/8(in8)
  octal_mux5/8(out7) -> bus_create7/8(in8)
  octal_mux5/7(out6) -> bus_create7/7(in7)
  octal_mux5/6(out5) -> bus_create7/6(in6)
  octal_mux5/5(out4) -> bus_create7/5(in5)
  octal_mux5/4(out3) -> bus_create7/4(in4)
  octal_mux5/3(out2) -> bus_create7/3(in3)
  octal_mux5/2(out1) -> bus_create7/2(in2)
  octal_mux5/1(out0) -> bus_create7/1(in1)
  [noise3] -> octal_mux5/4(n3)
  [noise2] -> octal_mux5/3(n2)
  [noise1] -> octal_mux5/2(n1)
  [noise0] -> octal_mux5/1(n0)
  [noise0] -> octal_mux6/1(n0)
  [noise1] -> octal_mux6/2(n1)
  [noise2] -> octal_mux6/3(n2)
  [noise3] -> octal_mux6/4(n3)
  octal_mux6/1(out0) -> bus_create8/1(in1)
  octal_mux6/2(out1) -> bus_create8/2(in2)
  octal_mux6/3(out2) -> bus_create8/3(in3)
  octal_mux6/4(out3) -> bus_create8/4(in4)
  octal_mux6/5(out4) -> bus_create8/5(in5)
  octal_mux6/6(out5) -> bus_create8/6(in6)
  octal_mux6/7(out6) -> bus_create8/7(in7)
  octal_mux6/8(out7) -> bus_create8/8(in8)
  octal_mux7/8(out7) -> bus_create9/8(in8)
  octal_mux7/7(out6) -> bus_create9/7(in7)
  octal_mux7/6(out5) -> bus_create9/6(in6)
  octal_mux7/5(out4) -> bus_create9/5(in5)
  octal_mux7/4(out3) -> bus_create9/4(in4)
  octal_mux7/3(out2) -> bus_create9/3(in3)
  octal_mux7/2(out1) -> bus_create9/2(in2)
  octal_mux7/1(out0) -> bus_create9/1(in1)
  [noise3] -> octal_mux7/4(n3)
  [noise2] -> octal_mux7/3(n2)
  [noise1] -> octal_mux7/2(n1)
  [noise0] -> octal_mux7/1(n0)
